simulink model "tvc_model_felix_rocket_simulation"  (R2024a)
settings: Solver=VariableStepAuto  StartTime=0.0  StopTime=20  RelTol=1e-3
libraries: simulink_extras x4, shared6dof x1, matrix_library x1
settings Model: Creator=Felix NIMY  LastModifiedBy=Felix NIMY

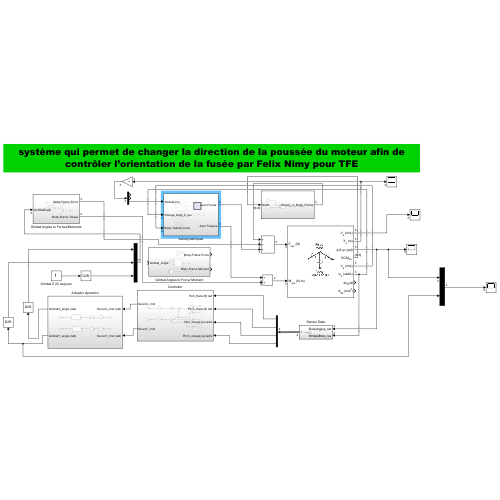
[thumbnail: Simulink's stored preview of the top-level diagram]
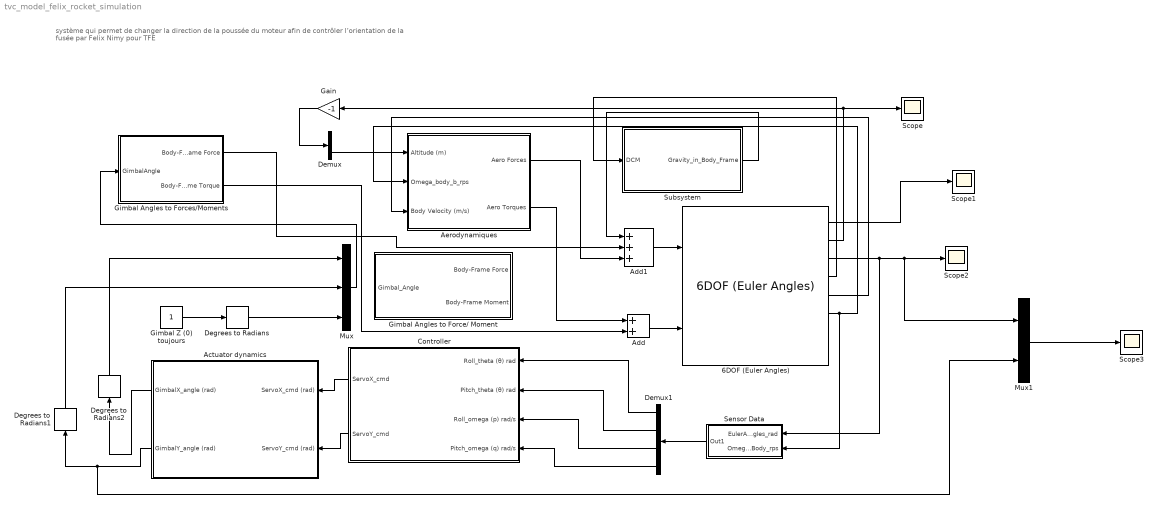
== system tvc_model_felix_rocket_simulation ==
  note: système qui permet de changer la direction de la poussée du moteur afin de contrôler l’orientation de la fusée par Felix Nimy pour TFE
  6DOF (Euler Angles) : shared6dof/6DOF (Euler Angles)  units=Metric (MKS)  mtype=Fixed  rep=Euler Angles  xme_0=[0 0 0]  Vm_0=[1 1 1]  eul_0=[0 0 0]  pm_0=[0 0 0]  mass_0=150  mass_e=0.5  mass_f=2.0  inertia=eye(3)  inertia_e=eye(3)  inertia_f=2*eye(3)  k_quat=1.0  vre_flag=on  abi_flag=off  aMode=0  xme_statename=''  Vm_statename=''  eul_statename=''  quat_statename=''  pm_statename=''  mass_statename=''
  Actuator dynamics : Subsystem
  Add : Sum
  Add1 : Sum  Inputs=+++
  Aerodynamiques : Subsystem
  Controller : Subsystem
  Degrees to Radians : simulink_extras/Transformations/Degrees to Radians
  Degrees to Radians1 : simulink_extras/Transformations/Degrees to Radians
  Degrees to Radians2 : simulink_extras/Transformations/Degrees to Radians
  Demux : Demux  Outputs=3
  Demux1 : Demux
  Gain : Gain  Gain=-1
  Gimbal Angles to Force/ Moment : Subsystem
  Gimbal Angles to Forces/Moments : Subsystem
  Gimbal Z (0) toujours : Constant
  Mux : Mux  Inputs=3
  Mux1 : Mux  Inputs=2
  Scope{,1..3} (4 alike) : Scope
  Sensor Data : Subsystem
  Subsystem : Subsystem
  wires:
  Add/1 -> 6DOF (Euler Angles)/2
  6DOF (Euler Angles)/5 -> Aerodynamiques/3(Body Velocity (m/s))
  6DOF (Euler Angles)/6 -> Aerodynamiques/2(Omega_body_b_rps), Sensor Data/2(OmegaBody_rps)
  6DOF (Euler Angles)/2 -> Gain/1, Scope/1
  Gain/1 -> Demux/1
  Demux/3 -> Aerodynamiques/1(Altitude (m))
  Add1/1 -> 6DOF (Euler Angles)/1
  Aerodynamiques/1("Aero Forces ") -> Add1/3
  Aerodynamiques/2(Aero Torques) -> Add/1
  6DOF (Euler Angles)/4 -> Subsystem/1(DCM)
  Subsystem/1(Gravity_in_Body_Frame) -> Add1/1
  6DOF (Euler Angles)/3 -> Mux1/1, Scope2/1, Sensor Data/1(EulerAngles_rad)
  Sensor Data/1(Out1) -> Demux1/1
  Demux1/1 -> Controller/1(Roll_theta (θ) rad)
  Demux1/2 -> Controller/2(Pitch_theta (θ) rad)
  Demux1/3 -> Controller/3(Roll_omega (p) rad/s)
  Demux1/4 -> Controller/4(Pitch_omega (q) rad/s)
  Controller/1(ServoX_cmd) -> Actuator dynamics/1(ServoX_cmd (rad))
  Controller/2(ServoY_cmd) -> Actuator dynamics/2(ServoY_cmd (rad))
  Gimbal Z (0) toujours/1 -> Degrees to Radians/1
  Degrees to Radians/1 -> Mux/3
  Gimbal Angles to Forces/Moments/2(Body-Frame Torque) -> Add/2
  Gimbal Angles to Forces/Moments/1(Body-Frame Force) -> Add1/2
  Actuator dynamics/2(GimbalY_angle (rad)) -> Mux1/2, Degrees to Radians1/1
  Degrees to Radians1/1 -> Mux/2
  Actuator dynamics/1(GimbalX_angle (rad)) -> Degrees to Radians2/1
  Degrees to Radians2/1 -> Mux/1
  Mux/1 -> Gimbal Angles to Forces/Moments/1(GimbalAngle)
  6DOF (Euler Angles)/1 -> Scope1/1
  Mux1/1 -> Scope3/1

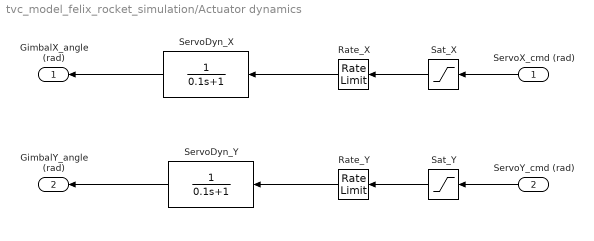
== system tvc_model_felix_rocket_simulation/Actuator dynamics ==
  ServoX_cmd (rad) : Inport
  ServoY_cmd (rad) : Inport  Port=2
  Rate_X : RateLimiter  RisingSlewLimit=deg2rad(60)  FallingSlewLimit=-deg2rad(60)  SampleTimeMode=inherited
  Rate_Y : RateLimiter  RisingSlewLimit=deg2rad(60)  FallingSlewLimit=-deg2rad(60)  SampleTimeMode=inherited
  Sat_X : Saturate  UpperLimit=deg2rad(5)  LowerLimit=-deg2rad(5)
  Sat_Y : Saturate  UpperLimit=deg2rad(5)  LowerLimit=-deg2rad(5)
  ServoDyn_X : TransferFcn  Denominator=[0.1 1]
  ServoDyn_Y : TransferFcn  Denominator=[0.1 1]
  GimbalX_angle (rad) : Outport
  GimbalY_angle (rad) : Outport  Port=2
  wires:
  ServoX_cmd (rad)/1 -> Sat_X/1
  Sat_X/1 -> Rate_X/1
  Rate_X/1 -> ServoDyn_X/1
  ServoDyn_X/1 -> GimbalX_angle (rad)/1
  Rate_Y/1 -> ServoDyn_Y/1
  Sat_Y/1 -> Rate_Y/1
  ServoY_cmd (rad)/1 -> Sat_Y/1
  ServoDyn_Y/1 -> GimbalY_angle (rad)/1

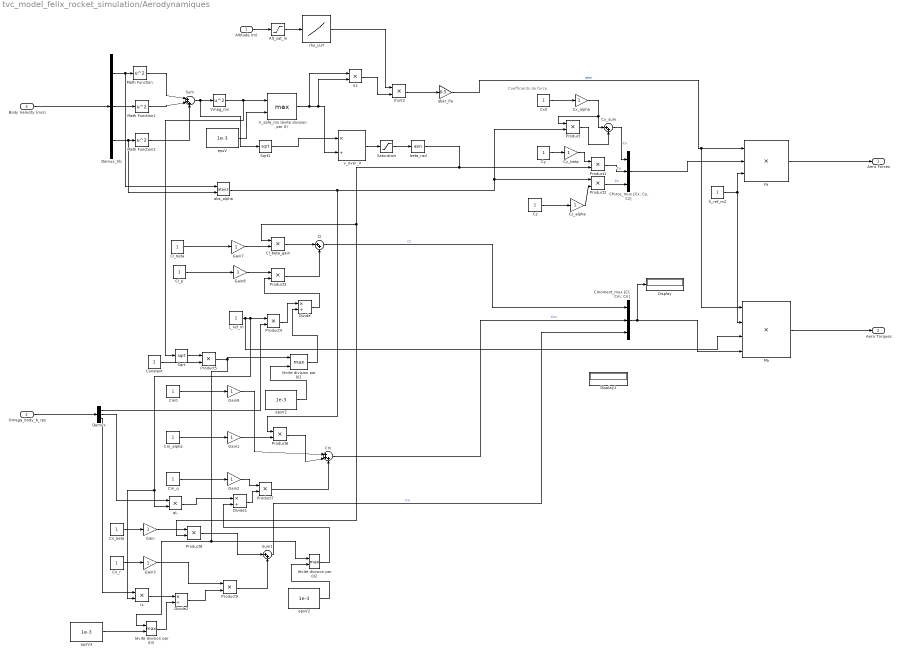
== system tvc_model_felix_rocket_simulation/Aerodynamiques ==
  note: Coefficients de force
  Altitude (m) : Inport
  Omega_body_b_rps : Inport  Port=2
  Body Velocity (m/s) : Inport  Port=3
  (évite division par 0)1 : MinMax  Function=max  Inputs=2
  (évite division par 0)2 : MinMax  Function=max  Inputs=2
  (évite division par 0)3 : MinMax  Function=max  Inputs=2
  Alt_sat_m : Saturate  UpperLimit=80000  LowerLimit=0
  Cforce_mux [Cx; Cy; Cz] : Mux  Inputs=3
  Cl : Sum  Inputs=|++
  Cl_beta : Constant
  Cl_beta_gain : Product
  Cl_p : Constant
  Cm : Sum  Inputs=|+++
  Cm0 : Constant
  Cm_alpha : Constant
  Cm_q : Constant
  Cmoment_mux [Cl; Cm; Cn] : Mux  Inputs=3
  Cn_beta : Constant
  Cn_r : Constant
  Constant : Constant  Value=2
  Cx0 : Constant
  Cx_alpha : Gain
  Cx_sum : Sum  Inputs=|++
  Cy : Constant
  Cy_beta : Gain
  Cz : Constant
  Cz_alpha : Gain
  Demux : Demux  Outputs=3
  Demux_Vb : Demux  Outputs=3
  Display : Display
  Display1 : Display
  Divide : Product  Inputs=*/
  Divide1 : Product  Inputs=*/
  Divide2 : Product  Inputs=*/
  Fa : Product  Inputs=3
  Gain{,1..3,7..9} (7 alike) : Gain
  L_ref_m : Constant
  Ma : Product  Inputs=4
  Math Function : Math  Operator=square
  Math Function1 : Math  Operator=square
  Math Function2 : Math  Operator=square
  Product{,1..9} (10 alike) : Product
  S_ref_m2 : Constant
  Saturation : Saturate  UpperLimit=1  LowerLimit=-1
  Sqrt : Sqrt
  Sqrt1 : Sqrt
  Sum : Sum  Inputs=|+++
  Sum1 : Sum  Inputs=|++
  V2 : Product
  V_safe_ms (évite division par 0) : MinMax  Function=max  Inputs=2
  Vmag_ms : Math  Operator=square
  abs_alpha : Trigonometry  Operator=atan2
  beta_rad : Trigonometry  Operator=asin
  epsV{,1..3} (4 alike) : Constant  Value=1e-3
  qL : Product
  qbar_Pa : Gain  Gain=0.5
  rL : Product
  rhoV2 : Product
  rho_LUT : Lookup_n-D  NumberOfTableDimensions=1  BreakpointsForDimension1=[-5:5]  Table=tanh([-5:5])  InternalRulePriority=Speed  RndMeth=Simplest
  v_over_V : Product  Inputs=*/
  "Aero Forces " : Outport
  Aero Torques : Outport  Port=2
  wires:
  Altitude (m)/1 -> Alt_sat_m/1
  Alt_sat_m/1 -> rho_LUT/1
  Body Velocity (m/s)/1 -> Demux_Vb/1
  Demux_Vb/1 -> abs_alpha/1, Math Function/1
  Demux_Vb/2 -> Math Function1/1
  Demux_Vb/3 -> abs_alpha/2, Math Function2/1
  Sum/1 -> Sqrt1/1, Vmag_ms/1
  Math Function/1 -> Sum/1
  Math Function1/1 -> Sum/2
  Math Function2/1 -> Sum/3
  Vmag_ms/1 -> Sqrt/1, V_safe_ms (évite division par 0)/1
  epsV/1 -> V_safe_ms (évite division par 0)/2
  V_safe_ms (évite division par 0)/1 -> V2/1, V2/2, v_over_V/2
  v_over_V/1 -> Saturation/1
  Saturation/1 -> beta_rad/1
  rho_LUT/1 -> rhoV2/1
  V2/1 -> rhoV2/2
  rhoV2/1 -> qbar_Pa/1
  Cx_alpha/1 -> Product/1, Cx_sum/1
  Cy/1 -> Cy_beta/1
  Cz/1 -> Cz_alpha/1
  Cx_sum/1 -> Cforce_mux [Cx; Cy; Cz]/1  "Cx"
  Cx0/1 -> Cx_alpha/1
  abs_alpha/1 -> Product6/1, Product/2, Product2/1
  Product/1 -> Cx_sum/2
  Cy_beta/1 -> Product1/1
  beta_rad/1 -> Product8/2, Cl_beta_gain/1, Product1/2
  Product1/1 -> Cforce_mux [Cx; Cy; Cz]/2  "Cy"
  Cz_alpha/1 -> Product2/2
  Product2/1 -> Cforce_mux [Cx; Cy; Cz]/3  "Cz"
  Omega_body_b_rps/1 -> Demux/1
  Cl_beta/1 -> Gain7/1
  Gain7/1 -> Cl_beta_gain/2
  Cl_p/1 -> Gain8/1
  Gain8/1 -> Product3/1
  L_ref_m/1 -> Ma/3, rL/2, qL/2, Product4/1
  Demux/1 -> Product4/2
  Constant/1 -> Product5/2
  Sqrt/1 -> Product5/1
  Product4/1 -> Divide/1
  Product5/1 -> (évite division par 0)3/1, (évite division par 0)2/1, (évite division par 0)1/1
  Divide/1 -> Product3/2
  Cl_beta_gain/1 -> Cl/1
  Product3/1 -> Cl/2
  Cm0/1 -> Gain9/1
  Cm_alpha/1 -> Gain1/1
  Cm_q/1 -> Gain2/1
  Gain1/1 -> Product6/2
  Demux/2 -> qL/1
  qL/1 -> Divide1/1
  Gain2/1 -> Product7/1
  Divide1/1 -> Product7/2
  Gain9/1 -> Cm/1
  Product6/1 -> Cm/2
  Product7/1 -> Cm/3
  Cn_beta/1 -> Gain/1
  Gain/1 -> Product8/1
  Cn_r/1 -> Gain3/1
  Demux/3 -> rL/1
  rL/1 -> Divide2/1
  Gain3/1 -> Product9/1
  Divide2/1 -> Product9/2
  Product8/1 -> Sum1/1
  Product9/1 -> Sum1/2
  Cl/1 -> Cmoment_mux [Cl; Cm; Cn]/1  "Cl"
  Cm/1 -> Cmoment_mux [Cl; Cm; Cn]/2  "Cm"
  Sum1/1 -> Cmoment_mux [Cl; Cm; Cn]/3  "Cn"
  qbar_Pa/1 -> Ma/1, Fa/1  "qbar"
  Cforce_mux [Cx; Cy; Cz]/1 -> Fa/2
  S_ref_m2/1 -> Fa/3, Ma/2
  Fa/1 -> "Aero Forces "/1
  Cmoment_mux [Cl; Cm; Cn]/1 -> Ma/4, Display/1
  Ma/1 -> Aero Torques/1
  Sqrt1/1 -> v_over_V/1
  epsV1/1 -> (évite division par 0)1/2
  (évite division par 0)1/1 -> Divide/2
  epsV2/1 -> (évite division par 0)2/2
  (évite division par 0)2/1 -> Divide1/2
  epsV3/1 -> (évite division par 0)3/2
  (évite division par 0)3/1 -> Divide2/2

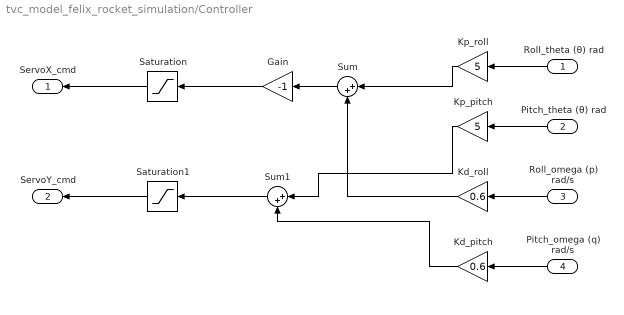
== system tvc_model_felix_rocket_simulation/Controller ==
  Roll_theta (θ) rad : Inport
  Pitch_theta (θ) rad : Inport  Port=2
  Roll_omega (p) rad/s : Inport  Port=3
  Pitch_omega (q) rad/s : Inport  Port=4
  Gain : Gain  Gain=-1
  Kd_pitch : Gain  Gain=0.6
  Kd_roll : Gain  Gain=0.6
  Kp_pitch : Gain  Gain=5
  Kp_roll : Gain  Gain=5
  Saturation : Saturate  UpperLimit=deg2rad(5)  LowerLimit=-deg2rad(5)
  Saturation1 : Saturate  UpperLimit=deg2rad(5)  LowerLimit=-deg2rad(5)
  Sum : Sum  Inputs=|++
  Sum1 : Sum  Inputs=|++
  ServoX_cmd : Outport
  ServoY_cmd : Outport  Port=2
  wires:
  Roll_theta (θ) rad/1 -> Kp_roll/1
  Kp_roll/1 -> Sum/1
  Kd_roll/1 -> Sum/2
  Sum/1 -> Gain/1
  Roll_omega (p) rad/s/1 -> Kd_roll/1
  Kp_pitch/1 -> Sum1/1
  Kd_pitch/1 -> Sum1/2
  Pitch_omega (q) rad/s/1 -> Kd_pitch/1
  Pitch_theta (θ) rad/1 -> Kp_pitch/1
  Gain/1 -> Saturation/1
  Sum1/1 -> Saturation1/1
  Saturation/1 -> ServoX_cmd/1
  Saturation1/1 -> ServoY_cmd/1

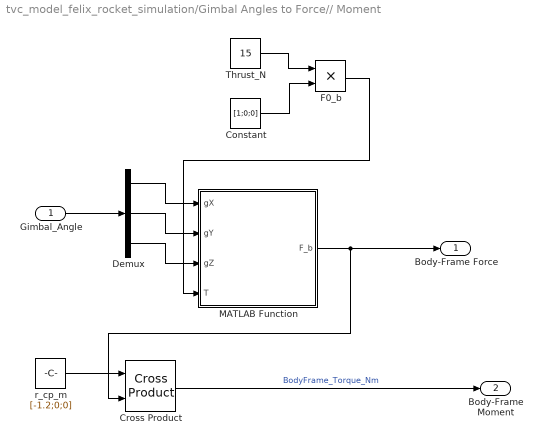
== system tvc_model_felix_rocket_simulation/Gimbal Angles to Force// Moment ==
  Gimbal_Angle : Inport
  Constant : Constant  Value=[1;0;0]
  Cross Product : matrix_library/Cross Product
  Demux : Demux  Outputs=3
  F0_b : Product
  MATLAB Function : MATLAB Function  TreatAsAtomicUnit=on
  Thrust_N : Constant  Value=15
  r_cp_m : Constant  Value=[-1.2;0;0]
  Body-Frame Force : Outport
  Body-Frame Moment : Outport  Port=2
  wires:
  Gimbal_Angle/1 -> Demux/1
  Thrust_N/1 -> F0_b/1
  Constant/1 -> F0_b/2
  Demux/1 -> MATLAB Function/1(gX)
  Demux/2 -> MATLAB Function/2(gY)
  Demux/3 -> MATLAB Function/3(gZ)
  MATLAB Function/1(F_b) -> Cross Product/2, Body-Frame Force/1
  r_cp_m/1 -> Cross Product/1
  Cross Product/1 -> Body-Frame Moment/1  "BodyFrame_Torque_Nm"
  F0_b/1 -> MATLAB Function/4(T)

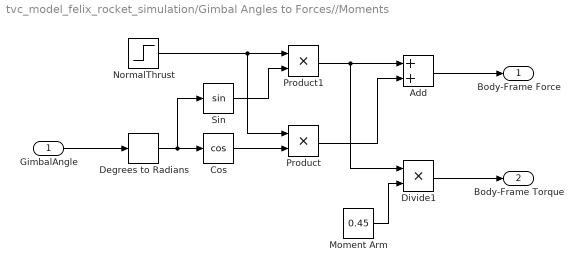
== system tvc_model_felix_rocket_simulation/Gimbal Angles to Forces//Moments ==
  GimbalAngle : Inport
  Add : Sum
  Cos : Trigonometry  Operator=cos
  Degrees to Radians : simulink_extras/Transformations/Degrees to Radians
  Divide1 : Product  Inputs=**
  "Moment Arm " : Constant  Value=0.45
  NormalThrust : Step  Time=2  Before=-15  After=0  SampleTime=0
  Product : Product  RndMeth=Zero
  Product1 : Product  RndMeth=Zero
  Sin : Trigonometry
  Body-Frame Force : Outport
  Body-Frame Torque : Outport  Port=2
  wires:
  Cos/1 -> Product/2
  NormalThrust/1 -> Product/1, Product1/1
  Sin/1 -> Product1/2
  Product1/1 -> Divide1/1, Add/1
  GimbalAngle/1 -> Degrees to Radians/1
  Degrees to Radians/1 -> Sin/1, Cos/1
  "Moment Arm "/1 -> Divide1/2
  Divide1/1 -> Body-Frame Torque/1
  Product/1 -> Add/2
  Add/1 -> Body-Frame Force/1

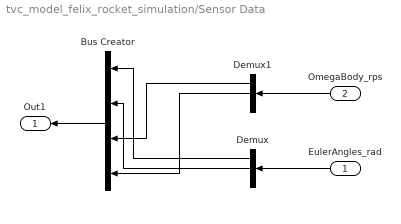
== system tvc_model_felix_rocket_simulation/Sensor Data ==
  EulerAngles_rad : Inport
  OmegaBody_rps : Inport  Port=2
  Bus Creator : BusCreator  Inputs=4
  Demux : Demux  Outputs=3
  Demux1 : Demux  Outputs=3
  Out1 : Outport
  wires:
  EulerAngles_rad/1 -> Demux/1
  OmegaBody_rps/1 -> Demux1/1
  Demux/1 -> Bus Creator/1
  Demux/2 -> Bus Creator/2
  Demux1/1 -> Bus Creator/3
  Demux1/2 -> Bus Creator/4
  Bus Creator/1 -> Out1/1

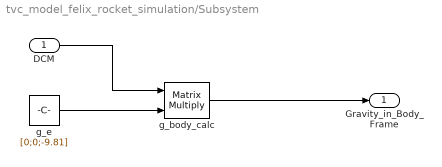
== system tvc_model_felix_rocket_simulation/Subsystem ==
  DCM : Inport
  g_body_calc : Product  Multiplication=Matrix(*)
  g_e : Constant  Value=[0;0;-9.81]
  Gravity_in_Body_Frame : Outport
  wires:
  g_e/1 -> g_body_calc/2
  DCM/1 -> g_body_calc/1
  g_body_calc/1 -> Gravity_in_Body_Frame/1

== matlab function tvc_model_felix_rocket_simulation/Gimbal Angles to Force// Moment/MATLAB Function ==
  data: gX input; F_b output; gY input; gZ input; T input
function F_b = GimbalRotation(gX,gY,gZ,T)
% Poussée nominale dans le repère corps
F0 = T;

% Rotations élémentaires (convention : X puis Y puis Z)
Rx = [1 0 0;
      0 cos(gX) -sin(gX);
      0 sin(gX)  cos(gX)];

Ry = [ cos(gY) 0 sin(gY);
       0 1 0;
      -sin(gY) 0 cos(gY)];

Rz = [cos(gZ) -sin(gZ) 0;
      sin(gZ)  cos(gZ) 0;
      0 0 1];


% Rotation totale (ordre à adapter selon ta convention)
R = Rz*Ry*Rx;

% Force de poussée orientée
F_b = R*F0;

end
